simulink subsystem "PIcontroller"  (R2020a)
settings: Solver=VariableStepAuto  StartTime=0.0  StopTime=10.0  RelTol=1e-3
undefined symbols (not defined in the file): Ki, Kp, Ts
settings Model: Creator=sonal  LastModifiedBy=sonal

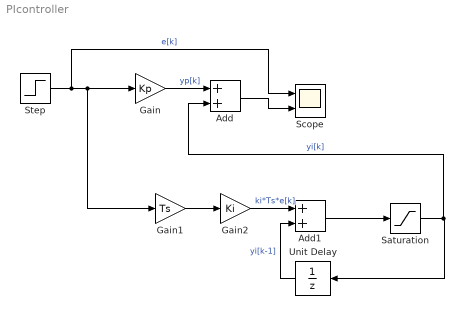
== system PIcontroller ==
  Add : Sum
  Add1 : Sum
  Gain : Gain  Gain=Kp
  Gain1 : Gain  Gain=Ts
  Gain2 : Gain  Gain=Ki
  Saturation : Saturate  UpperLimit=1  LowerLimit=-1
  Scope : Scope  NumInputPorts=2
  Step : Step  SampleTime=Ts
  Unit Delay : UnitDelay  SampleTime=-1  HasFrameUpgradeWarning=on
  wires:
  Add/1 -> Scope/2
  Gain/1 -> Add/1  "yp[k]"
  Step/1 -> Gain/1, Gain1/1, Scope/1  "e[k]"
  Gain2/1 -> Add1/1  "ki*Ts*e[k]"
  Unit Delay/1 -> Add1/2  "yi[k-1]"
  Saturation/1 -> Unit Delay/1, Add/2  "yi[k]"
  Add1/1 -> Saturation/1
  Gain1/1 -> Gain2/1
